simulink model "Obs_TP3_slx"  (R2020b)
settings: Solver=VariableStepAuto  StartTime=0.0  StopTime=inf  RelTol=1e-3
values from neighbouring files (symbols this model uses):
  AA = [0 1 0 0; 0 -1/0.31 981*pi/180 0; 0 0 0 1; 0 0 -144.1 -17.27]    [Sim_med.m]
  BB = [0; 0; 0; 61.8]    [Sim_med.m]
  CC = eye(4)    [Sim_med.m]
  DD = [0; 0; 0; 0]    [Sim_med.m]
  K2 = place(A2,-B2,[0.92, 0.91, 0.9, 0.89, 0.88])    [Obs_TP3.m]    (also in TP3_v2.m = place(A2,-B2, [0.876 + 0.01j, 0.876 - 0.01j, 0.895 + 0.01j, )
undefined symbols (not defined in the file or in its folder): serial
libraries: instrumentlib x2
settings Model: Creator=Dell  LastModifiedBy=Dell

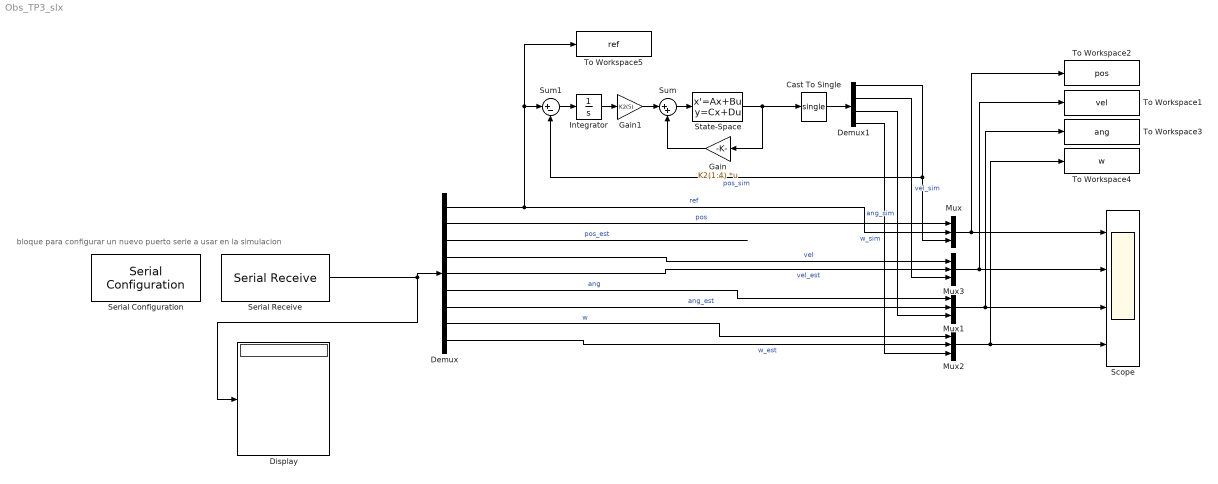
== system Obs_TP3_slx ==
  note: bloque para configurar un nuevo puerto serie a usar en la simulacion
  Cast To Single : DataTypeConversion  OutDataTypeStr=single
  Demux : Demux  Outputs=9
  Demux1 : Demux
  Display : Display
  Gain : Gain  Gain=K2(1:4)  Multiplication=Matrix(K*u)
  Gain1 : Gain  Gain=K2(5)
  Integrator : Integrator
  Mux{,1..3} (4 alike) : Mux  Inputs=3
  Scope : Scope  NumInputPorts=4
  Serial Configuration : instrumentlib/Serial Configuration  Priority=-200000  ComPortMenu=<Please select a port...>  ComPort=COM10  ObjConstructor=serial('COM10');  BaudRate=115200  DataBits=8  Parity=none  StopBits=1  FlowControl=none  Timeout=10  ByteOrder=LittleEndian
  Serial Receive : instrumentlib/Serial Receive  Priority=1  ComPortMenu=<Please select a port...>  ComPort=COM10  ObjConstructor=serial('COM10');  Header=abcd  Terminator=<none>  DataSize="[9  1]"  DataType=single  EnableBlockingMode=on  ActionDataUnavailable=Output last received value  CustomValue=0  SampleTime=0.02
  State-Space : StateSpace  A=AA  B=BB  C=CC  D=DD  InitialCondition=0
  Sum : Sum  Inputs=|++
  Sum1 : Sum  Inputs=|+-  OutDataTypeStr=double
  To Workspace1 : ToWorkspace  VariableName=vel  SampleTime=-1
      settings: Save2DSignal=2-D array (concatenate along first dimension)
  To Workspace2 : ToWorkspace  VariableName=pos  SampleTime=-1
      settings: Save2DSignal=2-D array (concatenate along first dimension)
  To Workspace3 : ToWorkspace  VariableName=ang  SampleTime=-1
      settings: Save2DSignal=2-D array (concatenate along first dimension)
  To Workspace4 : ToWorkspace  VariableName=w  SampleTime=-1
      settings: Save2DSignal=2-D array (concatenate along first dimension)
  To Workspace5 : ToWorkspace  VariableName=ref  SampleTime=-1
      settings: Save2DSignal=2-D array (concatenate along first dimension)
  wires:
  Demux/1 -> Mux/2, Sum1/1, To Workspace5/1  "ref"
  Serial Receive/1 -> Display/1, Demux/1
  Mux/1 -> To Workspace2/1, Scope/1
  Mux1/1 -> To Workspace3/1, Scope/3
  Demux/2 -> Mux/1  "pos"
  Demux/4 -> Mux3/1  "vel"
  Demux/6 -> Mux1/1  "ang"
  Demux/7 -> Mux1/2  "ang_est"
  Demux/8 -> Mux2/1  "w"
  Mux2/1 -> To Workspace4/1, Scope/4
  Demux/9 -> Mux2/2  "w_est"
  Mux3/1 -> To Workspace1/1, Scope/2
  Demux/3 -> ?  "pos_est"
  Demux/5 -> Mux3/2  "vel_est"
  Gain/1 -> Sum/2
  Gain1/1 -> Sum/1
  Sum/1 -> State-Space/1
  State-Space/1 -> Gain/1, Cast To Single/1
  Demux1/4 -> Mux2/3  "w_sim"
  Demux1/3 -> Mux1/3  "ang_sim"
  Demux1/2 -> Mux3/3  "vel_sim"
  Demux1/1 -> Mux/3, Sum1/2  "pos_sim"
  Cast To Single/1 -> Demux1/1
  Integrator/1 -> Gain1/1
  Sum1/1 -> Integrator/1
